simulink model "model3"  (R2015a)
settings: Solver=ode45  StartTime=0.0  StopTime=10.0  RelTol=1e-3
values from neighbouring files (symbols this model uses):
  A = [-((ms*g*l)/Kfric)  0          -(Is/Kfric) ... (first row only)    [balancin.m]
  B = [(Id/Is) -(Id/Is) 0]'    [balancin.m]
  C = [1 0 0 ... (first row only)    [balancin.m]
  D = [0 0 0]'    [balancin.m]
settings Model: Creator=Richa  LastModifiedBy=Richa

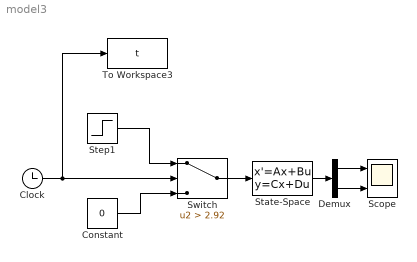
== system model3 ==
  Clock : Clock
  Constant : Constant  Value=0
  Demux : Demux  Outputs=2
  Scope : Scope  NumInputPorts=2
      settings: YMin=-5~-5  YMax=5~5
  State-Space : StateSpace  A=A  B=B  C=C  D=D  X0=0
  Step1 : Step  Time=3  Before=1405  After=0  SampleTime=0
  Switch : Switch  Criteria=u2 > Threshold  Threshold=2.92
  To Workspace3 : ToWorkspace  VariableName=t  SampleTime=-1
  wires:
  State-Space/1 -> Demux/1
  Clock/1 -> To Workspace3/1, Switch/2
  Step1/1 -> Switch/1
  Switch/1 -> State-Space/1
  Constant/1 -> Switch/3
  Demux/1 -> Scope/1
  Demux/2 -> Scope/2
